simulink model "COM_Prog_Rover"  (Simulink 7.8)
settings: Solver=FixedStepDiscrete  StartTime=0.0  StopTime=inf  FixedStep=ComMinSampleTime  RelTol=1e-3
undefined symbols (not defined in the file or in its folder): ComMinSampleTime, Gumstix
settings Model: Creator=Kjenab  LastModifiedBy=keynux  ExtModeTrigDuration=10000
settings SolverCC: PositivePriorityOrder=on
settings DataIOCC: SaveFormat=StructureWithTime
settings OptimizationCC: InitFltsAndDblsToZero=on  OptimizeModelRefInitCode=on  LifeSpan=Inf
settings DebuggingCC: SaveWithParameterizedLinksMsg=none  UnderspecifiedInitializationDetection=Simplified  MergeDetectMultiDrivingBlocksExec=error  FcnCallInpInsideContextMsg=Use local settings  FrameProcessingCompatibilityMsg=error
settings RTWCC: SystemTargetFile=ert.tlc  GenCodeOnly=on  GenerateMakefile=off  TemplateMakefile=ert_default_tmf  PostCodeGenCommand=packNGo(buildInfo, {'packType' 'hierarchical'})  Description=Embedded Coder  ProcessScript=ert_make_rtw_hook
settings CodeAppCC: IgnoreCustomStorageClasses=off
settings ERTTargetCC: TargetFunctionLibrary=C89/C90 (ANSI)  MultiwordLength=2048  GenerateSampleERTMain=on  ERTCustomFileTemplate=example_file_process.tlc  ConvertIfToSwitch=off  SuppressUnreachableDefaultCases=off

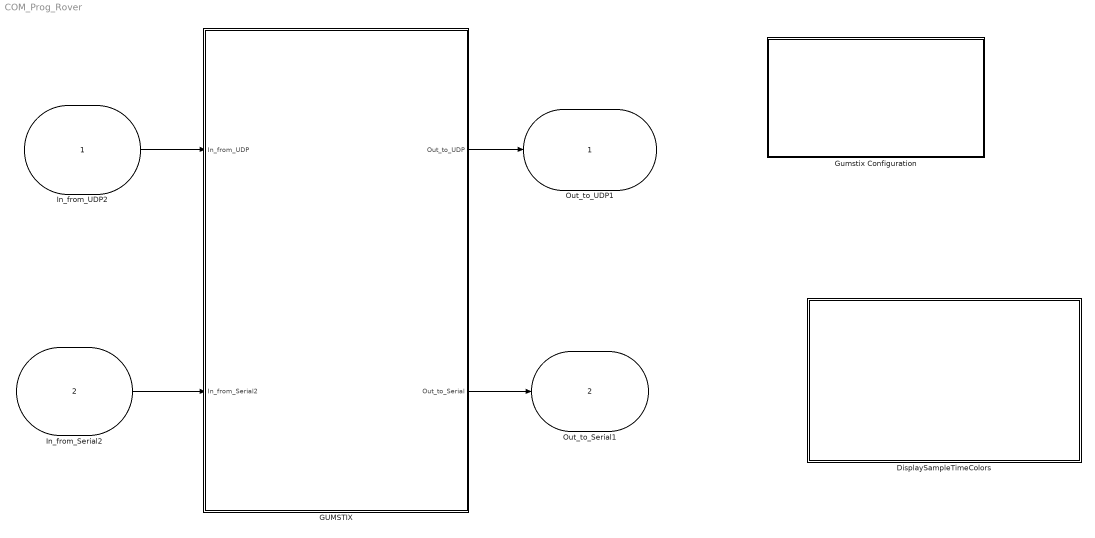
== system COM_Prog_Rover ==
  In_from_UDP2 : Inport  OutDataTypeStr=single  PortDimensions=Gumstix.UDP.Reception(1).NbData  SampleTime=Gumstix.UDP.Reception(1).SampleTime  mask{UDP_NbData=26, UDP_DataType=float32, UDP_remoteIPaddress='192.168.137.3', UDP_remotePort=2012, UDP_Interface=wlan0, UDP_localPort=2012, UDP_SampleTime=ComMinSampleTime, UDP_BlockingReception=OFF (try to read the n data), UDP_BlockingTimeOut=0.1}
      mask prompts: UDP_NbData "Number of Received Data"; UDP_DataType "UDP Data Type"; UDP_remoteIPaddress "Remote peer's IP address (IPv4)"; UDP_remotePort "Remote peer's Port (1023<port<65536)"; UDP_Interface "Local Interface to use"; UDP_localPort "Local Port (1023<port<65536)"; UDP_SampleTime "Reception Sample Time [s]"; UDP_BlockingReception "Blocking Reception"; UDP_BlockingTimeOut "Blocking Time Out [s]"
      mask init:
      | for i=1:1:8
      |     ProcessUDPInportMask_COM(gcb, i);
      | end
      mask StyleString: edit,popup(double64|float32|int32|unsigned int32|int16|unsigned int16|char8|unsigned char8),edit,edit,popup(wlan0|eth0),edit,edit,popup(ON (wait the n data until the Time Out)|OFF (try to read the n data)),edit
      mask CallbackString: ProcessUDPInportMask_COM(gcb, 1);|ProcessUDPInportMask_COM(gcb, 2);|ProcessUDPInportMask_COM(gcb, 3);|ProcessUDPInportMask_COM(gcb, 4);|ProcessUDPInportMask_COM(gcb, 5);|ProcessUDPInportMask_COM(gcb, 6);|ProcessUDPInportMask_COM(gcb, 7);|ProcessUDPInportMask_COM(gcb, 8);|ProcessUDPInportMask_COM(gcb, 9);
      mask Display: Display_UDP_Reception_Block;
  In_from_Serial2 : Inport  Port=2  OutDataTypeStr=uint8  PortDimensions=Gumstix.RS232.Reception(1).NbData  SampleTime=Gumstix.RS232.Reception(1).SampleTime  mask{RS232_NbData=6, RS232_DataType=unsigned char8, RS232_Port=/dev/ttyO0, RS232_BaudRate=115200, RS232_SampleTime=0.01, RS232_BlockingReception=OFF (try to read the n data), RS232_BlockingTimeOut=0.00022, RS232_StreamHeaderReception=1 byte, RS232_StreamHeaderValue=174, RS232_StartProtocol=SendStart -> WaitStart, RS232_StartTimeOut=100, RS232_StartStream=START, RS232_StopProtocol=None, RS232_StopTimeOut=100, RS232_StopStream=STOP}
      mask prompts: RS232_NbData "Number of Received Data"; RS232_DataType "RS232 Data Type"; RS232_Port "Serial Port"; RS232_BaudRate "BaudRate"; RS232_SampleTime "Reception Sample Time [s]"; RS232_BlockingReception "Blocking Reception"; RS232_BlockingTimeOut "Blocking Time Out [s]"; RS232_StreamHeaderReception "Stream Header"; RS232_StreamHeaderValue "Stream header value [0-255]"; RS232_StartProtocol "START Protocols"; RS232_StartTimeOut "Start Stream Waiting TimeOut [ms]"; RS232_StartStream "Start Message"; RS232_StopProtocol "STOP Protocols"; RS232_StopTimeOut "Stop Stream Waiting TimeOut [ms]"; RS232_StopStream "Stop Message"
      mask init:
      | for i=1:1:15
      |     ProcessRS232InportMask_COM(gcb, i);
      | end
      mask StyleString: edit,popup(double64|float32|int32|unsigned int32|int16|unsigned int16|char8|unsigned char8),popup(/dev/ttyO0|/dev/ttyO1|/dev/ttyO2|/dev/ttyO3|/dev/ttyO4|/dev/ttyO5|/dev/ttyO6|/dev/ttyO7|/dev/ttyO8|/dev/ttyO9|/dev/ttyO10|/dev/ttyO11|/dev/ttyO12|/dev/ttyO13|/dev/ttyO14|/dev/ttyO15|/dev/ttyUSB0|/dev/ttyUSB1),popup(50|75|110|134|150|200|300|600|1200|1800|2400|4800|9600|19200|38400|57600|115200|230400|460800|576000|921600|1000000|1152000|1500000|2000000|2500000|3000000|3500000|4000000),edit,popup(ON (wait the n data)|OFF (try to read the n data)),edit,popup(None|1 byte),edit,popup(WaitStart -> SendStart|SendStart -> WaitStart|None),edit,edit,popup(WaitStop -> SendStop|SendStop -> WaitStop|None),edit,edit
      mask CallbackString:
      | ProcessRS232InportMask_COM(gcb, 1);
      | |ProcessRS232InportMask_COM(gcb, 2);
      | |ProcessRS232InportMask_COM(gcb, 3);
      | |ProcessRS232InportMask_COM(gcb, 4);
      | |ProcessRS232InportMask_COM(gcb, 5);
      | |ProcessRS232InportMask_COM(gcb, 6);
      | |ProcessRS232InportMask_COM(gcb, 7);|ProcessRS232InportMask_COM(gcb, 8);|ProcessRS232InportMask_COM(gcb, 9);|ProcessRS232InportMask_COM(gcb, 10);
      | |ProcessRS232InportMask_COM(gcb, 11);
      | |ProcessRS232InportMask_COM(gcb, 12);
      | |ProcessRS232InportMask_COM(gcb, 13);
      | |ProcessRS232InportMask_COM(gcb, 14);
      | |ProcessRS232InportMask_COM(gcb, 15);
      mask TabNameString: Reception,Reception,Reception,Reception,Reception,Reception,Reception,Header and Synchro Protocol,Header and Synchro Protocol,Header and Synchro Protocol,Header and Synchro Protocol,Header and Synchro Protocol,Header and Synchro Protocol,Header and Synchro Protocol,Header and Synchro Protocol
      mask Display: Display_RS232_Reception_Block;
  DisplaySampleTimeColors : Subsystem  mask{SampleTime_1=0.002, SampleTime_2=0.004, SampleTime_3=0.01}
      settings: OpenFcn=DisplaySampleTimeColors;
      mask Display:
      | ColorOrder = {'red', 'green', 'blue', 'orange', 'magenta', 'gray', 'cyan', 'yellow'};
      | MyMaskPrompt =  get_param(gcb, 'MaskPrompts');
      | Nb_Prompt = length(MyMaskPrompt);
      | color('black');
      | disp(sprintf('Display Sample Time Colors\n(double-click)'));
      | offset = '\n\n';
      | for nb_line=1:1:Nb_Prompt-1
      |     offset = [offset '\n\n'];
      |     color(ColorOrder{nb_line});
      |     currentSampleTime = eval(['SampleTime_' num2str(nb_line)]);
      |     if (currentSampleTime == '0') % their is continous states
      |         eval(['disp([sprintf(offset) ''SampleTime_'' num2str(nb_line) '' (fundamental solver step) '' '' = '' num2str(SampleTime_' num2str(nb_line+1) ') ''[s] (continous states)'']);']);
      |     else
      |         if (nb_line == 1)
      |             eval(['disp([sprintf(offset) ''SampleTime_'' num2str(nb_line) '' (fundamental solver step) '' '' = '' num2str(SampleTime_' num2str(nb_line) ') ''[s]'']);']);
      |         else
      |             eval(['disp([sprintf(offset) ''SampleTime_'' num2str(nb_line) '' = '' num2str(SampleTime_' num2str(nb_line) ') ''[s]'']);']);
      |         end
      |     end
      | end
      | color('black');
      | disp([sprintf(offset) sprintf('\n\nMore than 1 SampleTime (inside)')]);
  GUMSTIX : Subsystem
  Gumstix Configuration : Subsystem  mask{TimeSynchro=Internal Clock, RS232_InterruptSource=/dev/ttyO0, UDP_InterruptSource=wlan0, PrintfMode=off, FprintfMode=off, TimeLoggerMode=off, PrintfTimeMode=off, FprintfTimeMode=off, TaskingMode=Multi-Tasking, SchedPolicy=SCHED_RR        (Real-Time Scheduler), MaxTaskPriority=96, RTsystem=PREEMPT-RT}
      mask prompts: TimeSynchro "Time Scheduler"; RS232_InterruptSource "RS232 Interrupt Source"; UDP_InterruptSource "UDP Interrupt Source"; PrintfMode "Verbose mode activated in the Gumstix console"; FprintfMode "Verbose mode logged in a file (onto Gumstix)"; TimeLoggerMode "Time logger mode activated (log time exec of each task)"; PrintfTimeMode "Execution time plotted in the Gumstix console"; FprintfTimeMode "Execution time logged in a file (onto Gumstix)"; TaskingMode "Tasking Mode"; SchedPolicy "Scheduler Policy"; MaxTaskPriority "Maximum Task Priority [1-99]"; RTsystem "RT system"
      mask init:
      | for i=1:1:12
      |     ProcessConfigMask_COM(gcb, i);
      | end
      mask StyleString: popup(RS232 Reception|Internal Clock|UDP Reception),popup(/dev/ttyS0|/dev/ttyS1|/dev/ttyS2|/dev/ttyS3|/dev/ttyO0|/dev/ttyO1|/dev/ttyO2|/dev/ttyO3),popup(wlan0|eth0),popup(off|on),popup(off|on),popup(off|on),popup(off|on),popup(off|on),popup(Multi-Tasking|Single-Tasking),popup(SCHED_FIFO     (Real-Time Scheduler)|SCHED_RR        (Real-Time Scheduler)|SCHED_OTHER (NO Real-Time Scheduler)),edit,popup(PREEMPT-RT|XENOMAI)
      mask CallbackString: ProcessConfigMask_COM(gcb, 1);|ProcessConfigMask_COM(gcb, 2);|ProcessConfigMask_COM(gcb, 3);|ProcessConfigMask_COM(gcb, 4);|ProcessConfigMask_COM(gcb, 5);|ProcessConfigMask_COM(gcb, 6);|ProcessConfigMask_COM(gcb, 7);|ProcessConfigMask_COM(gcb, 8);|ProcessConfigMask_COM(gcb, 9);|ProcessConfigMask_COM(gcb, 10);|ProcessConfigMask_COM(gcb, 11);|ProcessConfigMask_COM(gcb, 12);
      mask TabNameString: TimeScheduler,TimeScheduler,TimeScheduler,Input-Ouput Verbose,Input-Ouput Verbose,Input-Ouput Verbose,Timing Debug,Timing Debug,TimeScheduler,TimeScheduler,TimeScheduler,TimeScheduler
      mask Display: image(imread('Configuration_v2.jpg'));
  Out_to_UDP1 : Outport  OutDataTypeStr=single  PortDimensions=Gumstix.UDP.Emission(1).NbData  SampleTime=Gumstix.UDP.Emission(1).SampleTime  mask{UDP_NbData=20, UDP_DataType=float32, UDP_RemoteIPaddress='192.168.137.3', UDP_RemotePort=2012, UDP_Interface=wlan0, UDP_LocalPort=2012, UDP_SampleTime=ComMinSampleTime}
      mask prompts: UDP_NbData "Number of Sent Data"; UDP_DataType "UDP Data Type"; UDP_RemoteIPaddress "remote peer's IP address (IPv4)"; UDP_RemotePort "remote peer's Port (1023<port<65536)"; UDP_Interface "Local Interface to use for UDP"; UDP_LocalPort "Local port to use"; UDP_SampleTime "Emission Sample Time [s]"
      mask init:
      | for i=1:1:7
      |     ProcessUDPOutportMask_COM(gcb, i);
      | end
      mask StyleString: edit,popup(double64|float32|int32|unsigned int32|int16|unsigned int16|char8|unsigned char8),edit,edit,popup(wlan0|eth0),edit,edit
      mask CallbackString: ProcessUDPOutportMask_COM(gcb, 1);|ProcessUDPOutportMask_COM(gcb, 2);|ProcessUDPOutportMask_COM(gcb, 3);|ProcessUDPOutportMask_COM(gcb, 4);|ProcessUDPOutportMask_COM(gcb, 5);|ProcessUDPOutportMask_COM(gcb, 6);|ProcessUDPOutportMask_COM(gcb, 7);
      mask Display: Display_UDP_Emission_Block;
  Out_to_Serial1 : Outport  Port=2  OutDataTypeStr=uint16  PortDimensions=Gumstix.RS232.Emission(1).NbData  SampleTime=Gumstix.RS232.Emission(1).SampleTime  mask{RS232_NbData=1, RS232_DataType=unsigned int16, RS232_Port=/dev/ttyO0, RS232_BaudRate=115200, RS232_SampleTime=0.01, RS232_StreamHeaderReception=1 byte, RS232_StreamHeaderValue=174, RS232_StartProtocol=SendStart -> WaitStart, RS232_StartTimeOut=100, RS232_StartStream=START, RS232_StopProtocol=None, RS232_StopTimeOut=100, RS232_StopStream=STOP}
      mask prompts: RS232_NbData "Number of Sent Data"; RS232_DataType "RS232 Data Type"; RS232_Port "Serial Port"; RS232_BaudRate "BaudRate"; RS232_SampleTime "Sample Time [s]"; RS232_StreamHeaderReception "Stream Header"; RS232_StreamHeaderValue "Stream header value [0-255]"; RS232_StartProtocol "RS232 Start Protocol"; RS232_StartTimeOut "Start Stream Waiting TimeOut [ms]"; RS232_StartStream "Start Message"; RS232_StopProtocol "RS232 Stop Protocol"; RS232_StopTimeOut "Stop Stream Waiting TimeOut [ms]"; RS232_StopStream "Stop Message"
      mask init:
      | for i=1:1:13
      |     ProcessRS232OutportMask_COM(gcb, i);
      | end
      mask StyleString: edit,popup(double64|float32|int32|unsigned int32|int16|unsigned int16|char8|unsigned char8),popup(/dev/ttyO0|/dev/ttyO1|/dev/ttyO2|/dev/ttyO3|/dev/ttyO4|/dev/ttyO5|/dev/ttyO6|/dev/ttyO7|/dev/ttyO8|/dev/ttyO9|/dev/ttyO10|/dev/ttyO11|/dev/ttyO12|/dev/ttyO13|/dev/ttyO14|/dev/ttyO15|/dev/ttyUSB0|/dev/ttyUSB1),popup(50|75|110|134|150|200|300|600|1200|1800|2400|4800|9600|19200|38400|57600|115200|230400|460800|576000|921600|1000000|1152000|1500000|2000000|2500000|3000000|3500000|4000000),edit,popup(None|1 byte),edit,popup(WaitStart -> SendStart|SendStart -> WaitStart|None),edit,edit,popup(WaitStop -> SendStop|SendStop -> WaitStop|None),edit,edit
      mask CallbackString:
      | ProcessRS232OutportMask_COM(gcb, 1);
      | |ProcessRS232OutportMask_COM(gcb, 2);
      | |ProcessRS232OutportMask_COM(gcb, 3);
      | |ProcessRS232OutportMask_COM(gcb, 4);
      | |ProcessRS232OutportMask_COM(gcb, 5);
      | |ProcessRS232OutportMask_COM(gcb, 6);|ProcessRS232OutportMask_COM(gcb, 7);|ProcessRS232OutportMask_COM(gcb, 8);|ProcessRS232OutportMask_COM(gcb, 9);|ProcessRS232OutportMask_COM(gcb, 10);|ProcessRS232OutportMask_COM(gcb, 11);|ProcessRS232OutportMask_COM(gcb, 12);|ProcessRS232OutportMask_COM(gcb, 13);
      mask TabNameString: Emission,Emission,Emission,Emission,Emission,Header and Synchro Protocol,Header and Synchro Protocol,Header and Synchro Protocol,Header and Synchro Protocol,Header and Synchro Protocol,Header and Synchro Protocol,Header and Synchro Protocol,Header and Synchro Protocol
      mask Display: Display_RS232_Emission_Block;
  wires:
  GUMSTIX/1(Out_to_UDP) -> Out_to_UDP1/1
  In_from_UDP2/1 -> GUMSTIX/1(In_from_UDP)
  In_from_Serial2/1 -> GUMSTIX/2("In_from_Serial2 ")
  GUMSTIX/2(Out_to_Serial) -> Out_to_Serial1/1

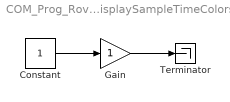
== system COM_Prog_Rover/DisplaySampleTimeColors ==
  Constant : Constant  OutDataTypeStr=uint8
  Gain : Gain
  Terminator : Terminator
  wires:
  Constant/1 -> Gain/1
  Gain/1 -> Terminator/1

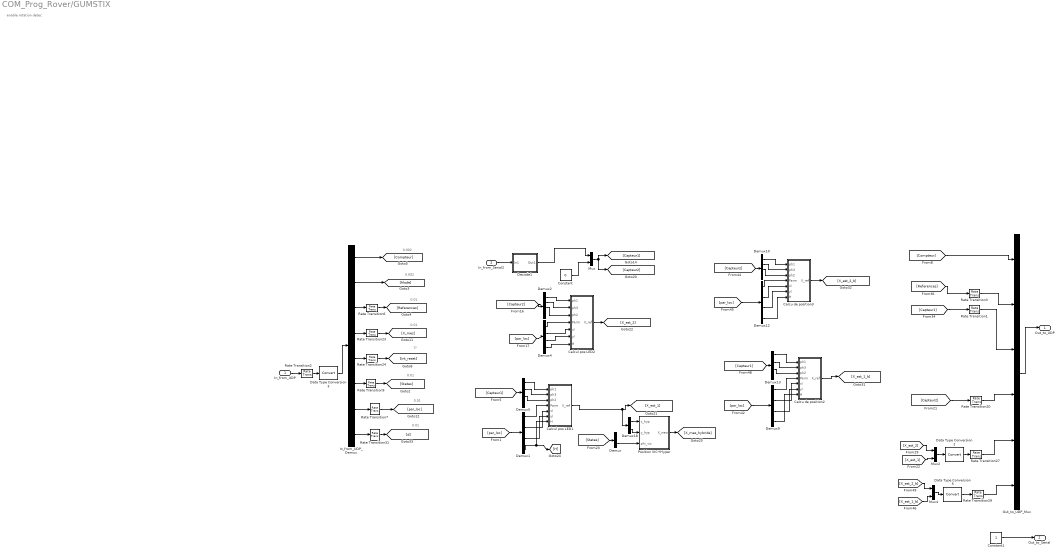
== system COM_Prog_Rover/GUMSTIX ==
  note: enable rotation detec
  note: 0.002
  note: 0.002
  note: 0.01
  note: 0.01
  note: 0.01
  note: 0.01
  note: 0.01
  note: ??
  In_from_UDP : Inport
  "In_from_Serial2 " : Inport  Port=2
  Calcu de position2 : MATLAB Function  TreatAsAtomicUnit=on
  Calcu de position3 : MATLAB Function  TreatAsAtomicUnit=on
  Calcul pos LED1 : MATLAB Function  TreatAsAtomicUnit=on
  Calcul pos LED2 : MATLAB Function  TreatAsAtomicUnit=on
  Constant : Constant  Value=0  OutDataTypeStr=Inherit: Inherit via back propagation  SampleTime=0.01
  Constant1 : Constant  OutDataTypeStr=Inherit: Inherit via back propagation  SampleTime=0.01
  Data Type Conversion2 : DataTypeConversion
  Data Type Conversion3 : DataTypeConversion
  Data Type Conversion5 : DataTypeConversion
  Decode1 : Subsystem
  Demux : Demux  Outputs=[2 1]
  Demux{1,4,9,12} (4 alike) : Demux  Outputs=[10 1 1 1]
  Demux10 : Demux  Outputs=[ 1 1 1 1]
  Demux13 : Demux  Outputs=[ 1 1 1 1]
  Demux18 : Demux  Outputs=[1 1]
  Demux2 : Demux  Outputs=[1 1 1 1]
  Demux5 : Demux  Outputs=[1 1 1 1]
  In_from_UDP_Demux : Demux  Outputs=[1 1 3 3 1 3 13 1]
  Mux : Mux  Inputs=2
  Mux2 : Mux  Inputs=2
  Mux4 : Mux  Inputs=2
  Out_to_UDP_Mux : Mux  Inputs=[1 3 4 4 4 4]
  Position VIC+Hyper : MATLAB Function  TreatAsAtomicUnit=on
  Rate Transition{1,3,20,27,29} (5 alike) : RateTransition
  Rate Transition2 : RateTransition  Deterministic=off
  Rate Transition{6..7,9,23,31} (5 alike) : RateTransition  Deterministic=off  OutPortSampleTime=Ts_control
  Rate Transition24 : RateTransition  Deterministic=off
  Out_to_UDP : Outport
  Out_to_Serial : Outport  Port=2
  wires:
  In_from_UDP/1 -> Rate Transition2/1
  Rate Transition2/1 -> Data Type Conversion3/1
  Data Type Conversion3/1 -> In_from_UDP_Demux/1
  In_from_UDP_Demux/1 -> [Compteur]
  In_from_UDP_Demux/2 -> [Mode]
  Rate Transition9/1 -> [States]
  [References] -> Rate Transition3/1
  Rate Transition6/1 -> [References]
  Rate Transition23/1 -> [X_mes]
  Rate Transition24/1 -> [Int_reset]
  Rate Transition3/1 -> Out_to_UDP_Mux/2
  Demux1/1 -> Calcul pos LED1/4(Parm)
  Rate Transition7/1 -> [par_loc]
  Demux1/2 -> Calcul pos LED1/5(xl)
  Demux1/3 -> Calcul pos LED1/6(yl)
  Demux1/4 -> [H], Calcul pos LED1/7(H)
  [Capteur2] -> Rate Transition20/1
  [par_loc] -> Demux4/1
  Demux4/1 -> Calcul pos LED2/4(Parm)
  Demux4/2 -> Calcul pos LED2/5(xl)
  Demux4/3 -> Calcul pos LED2/6(yl)
  Demux4/4 -> Calcul pos LED2/7(H)
  [Capteur2] -> Demux2/1
  Calcul pos LED2/1(X_ref) -> [X_est_2]
  [Compteur] -> Out_to_UDP_Mux/1
  Out_to_UDP_Mux/1 -> Out_to_UDP/1
  [X_est_2] -> Mux2/1
  Mux2/1 -> Data Type Conversion2/1
  Data Type Conversion2/1 -> Rate Transition27/1
  [X_est_1] -> Mux2/2
  Position VIC+Hyper/1(X_new) -> [X_mes_hybride]
  [Capteur1] -> Rate Transition1/1
  [States] -> Demux/1
  Demux9/1 -> Calcu de position2/4(Parm)
  [par_loc] -> Demux9/1
  Demux9/2 -> Calcu de position2/5(xl)
  Demux9/3 -> Calcu de position2/6(yl)
  Demux9/4 -> Calcu de position2/7(H)
  [Capteur1] -> Demux13/1
  [par_loc] -> Demux12/1
  Demux12/1 -> Calcu de position3/4(Parm)
  Demux12/2 -> Calcu de position3/5(xl)
  Demux12/3 -> Calcu de position3/6(yl)
  Demux12/4 -> Calcu de position3/7(H)
  [Capteur2] -> Demux10/1
  Calcu de position3/1(X_ref) -> [X_est_2_b]
  Demux10/1 -> Calcu de position3/1(ph1)
  Demux10/2 -> Calcu de position3/2(ph3)
  Demux10/3 -> Calcu de position3/3(ph2)
  Demux13/1 -> Calcu de position2/1(ph1)
  Demux13/2 -> Calcu de position2/2(ph3)
  Demux13/3 -> Calcu de position2/3(ph2)
  Calcul pos LED1/1(X_ref) -> Demux18/1, [X_est_1]
  [X_est_2_b] -> Mux4/1
  Mux4/1 -> Data Type Conversion5/1
  Data Type Conversion5/1 -> Rate Transition29/1
  [X_est_1_b] -> Mux4/2
  Rate Transition31/1 -> [d]
  Demux18/2 -> Position VIC+Hyper/2(y_hyp)
  Demux18/1 -> Position VIC+Hyper/1(x_hyp)
  Demux/2 -> Position VIC+Hyper/3(phi_vic)
  [par_loc] -> Demux1/1
  [Capteur1] -> Demux5/1
  Calcu de position2/1(X_ref) -> [X_est_1_b]
  Rate Transition1/1 -> Out_to_UDP_Mux/3
  In_from_UDP_Demux/3 -> Rate Transition6/1
  In_from_UDP_Demux/4 -> Rate Transition23/1
  In_from_UDP_Demux/5 -> Rate Transition24/1
  In_from_UDP_Demux/6 -> Rate Transition9/1
  In_from_UDP_Demux/7 -> Rate Transition7/1
  In_from_UDP_Demux/8 -> Rate Transition31/1
  Rate Transition20/1 -> Out_to_UDP_Mux/4
  Rate Transition27/1 -> Out_to_UDP_Mux/5
  Rate Transition29/1 -> Out_to_UDP_Mux/6
  "In_from_Serial2 "/1 -> Decode1/1(In1)
  Decode1/1(Out1) -> Mux/1
  Constant/1 -> Mux/2
  Mux/1 -> [Capteur1], [Capteur2]
  Demux2/1 -> Calcul pos LED2/1(ph1)
  Demux2/2 -> Calcul pos LED2/2(ph3)
  Demux2/3 -> Calcul pos LED2/3(ph2)
  Demux5/1 -> Calcul pos LED1/1(ph1)
  Demux5/2 -> Calcul pos LED1/2(ph3)
  Demux5/3 -> Calcul pos LED1/3(ph2)
  Constant1/1 -> Out_to_Serial/1

== system COM_Prog_Rover/Gumstix Configuration ==

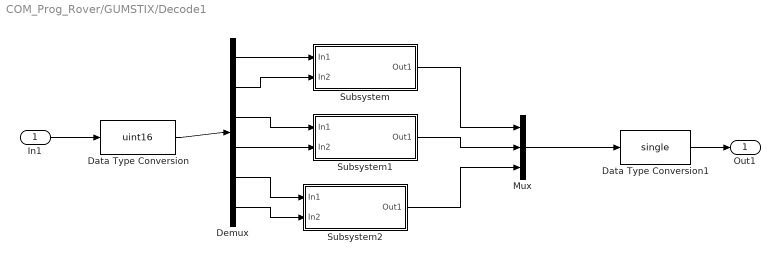
== system COM_Prog_Rover/GUMSTIX/Decode1 ==
  In1 : Inport
  Data Type Conversion : DataTypeConversion  OutDataTypeStr=uint16
  Data Type Conversion1 : DataTypeConversion  OutDataTypeStr=single
  Demux : Demux  Outputs=6
  Mux : Mux  Inputs=3
  Subsystem : Subsystem
  Subsystem1 : Subsystem
  Subsystem2 : Subsystem
  Out1 : Outport
  wires:
  Data Type Conversion1/1 -> Out1/1
  In1/1 -> Data Type Conversion/1
  Data Type Conversion/1 -> Demux/1
  Demux/1 -> Subsystem/1(In1)
  Demux/2 -> Subsystem/2(In2)
  Demux/3 -> Subsystem1/1(In1)
  Demux/4 -> Subsystem1/2(In2)
  Demux/5 -> Subsystem2/1(In1)
  Demux/6 -> Subsystem2/2(In2)
  Subsystem/1(Out1) -> Mux/1
  Subsystem1/1(Out1) -> Mux/2
  Subsystem2/1(Out1) -> Mux/3
  Mux/1 -> Data Type Conversion1/1

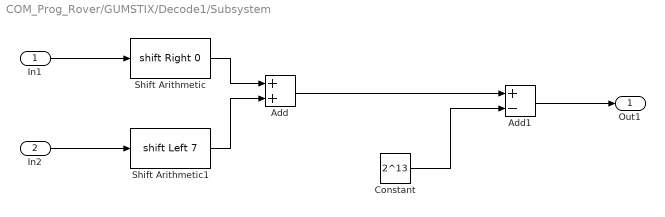
== system COM_Prog_Rover/GUMSTIX/Decode1/Subsystem ==
  In1 : Inport
  In2 : Inport  Port=2
  Add : Sum
  Add1 : Sum  Inputs=+-
  Constant : Constant  Value=2^13  OutDataTypeStr=uint16  SampleTime=-1
  Shift Arithmetic : ArithShift  BitShiftDirection=Right
  Shift Arithmetic1 : ArithShift  BitShiftNumber=7  BitShiftDirection=Left
  Out1 : Outport
  wires:
  In1/1 -> Shift Arithmetic/1
  In2/1 -> Shift Arithmetic1/1
  Shift Arithmetic/1 -> Add/1
  Shift Arithmetic1/1 -> Add/2
  Add/1 -> Add1/1
  Constant/1 -> Add1/2
  Add1/1 -> Out1/1

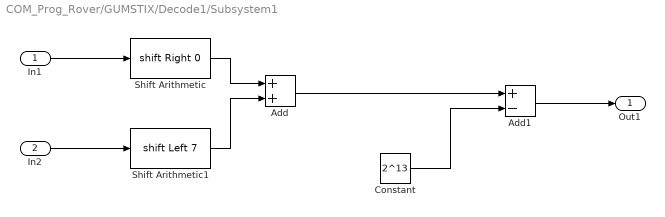
== system COM_Prog_Rover/GUMSTIX/Decode1/Subsystem1 ==
  In1 : Inport
  In2 : Inport  Port=2
  Add : Sum
  Add1 : Sum  Inputs=+-
  Constant : Constant  Value=2^13  OutDataTypeStr=uint16  SampleTime=-1
  Shift Arithmetic : ArithShift  BitShiftDirection=Right
  Shift Arithmetic1 : ArithShift  BitShiftNumber=7  BitShiftDirection=Left
  Out1 : Outport
  wires:
  In1/1 -> Shift Arithmetic/1
  In2/1 -> Shift Arithmetic1/1
  Shift Arithmetic/1 -> Add/1
  Shift Arithmetic1/1 -> Add/2
  Add/1 -> Add1/1
  Constant/1 -> Add1/2
  Add1/1 -> Out1/1

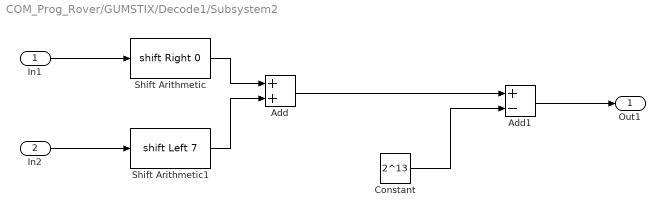
== system COM_Prog_Rover/GUMSTIX/Decode1/Subsystem2 ==
  In1 : Inport
  In2 : Inport  Port=2
  Add : Sum
  Add1 : Sum  Inputs=+-
  Constant : Constant  Value=2^13  OutDataTypeStr=uint16  SampleTime=-1
  Shift Arithmetic : ArithShift  BitShiftDirection=Right
  Shift Arithmetic1 : ArithShift  BitShiftNumber=7  BitShiftDirection=Left
  Out1 : Outport
  wires:
  In1/1 -> Shift Arithmetic/1
  In2/1 -> Shift Arithmetic1/1
  Shift Arithmetic/1 -> Add/1
  Shift Arithmetic1/1 -> Add/2
  Add/1 -> Add1/1
  Constant/1 -> Add1/2
  Add1/1 -> Out1/1

== matlab function GUMSTIX/Calcul pos LED2 ==
  data: ph1 input double; ph3 input double; X_ref output double; ph2 input double; Parm input double; xl input double; yl input double; H input double
function X_ref = position(ph1, ph3, ph2, Parm, xl, yl, H)   %xl,yl,H qre position of LED1
trd = pi/180;
tr2 = (ph1-ph2)/(ph1+ph2);
tr1 = (((ph1+ph2)/2)-ph3)/(((ph1+ph2)/2)+ph3);
%x = H*tan(trd*(a1*tr1+b1));
%y = H*tan(trd*(a2*tr2+b2));
% x = H.*tan(trd.*(Parm(1).*tr1 + Parm(2).*tr1.^2+ Parm(3).*tr2+Parm(4) ));
% y = H.*tan(trd.*(Parm(5).*tr2 + Parm(6).*tr2.^2+Parm(7).*tr1 + Parm(8)));
x = H.*tan(trd.*(Parm(1).*tr1 + Parm(2).*tr1.^2+ Parm(3).*tr2+  Parm(4).*tr2.^2+Parm(5) ));
y = H.*tan(trd.*(Parm(6).*tr2 + Parm(7).*tr2.^2+Parm(8).*tr1 + Parm(9).*tr1.^2+Parm(10)));
X_ref = [x,y];
end

== matlab function GUMSTIX/Calcu de position2 ==
  data: ph1 input double; ph3 input double; X_ref output double; ph2 input double; Parm input double; xl input double; yl input double; H input double
function X_ref = position(ph1, ph3, ph2, Parm, xl, yl, H)
trd = pi/180;
tr2 = (ph1-ph2)/(ph1+ph2);
tr1 = (((ph1+ph2)/2)-ph3)/(((ph1+ph2)/2)+ph3);
%x = H*tan(trd*(a1*tr1+b1));
%y = H*tan(trd*(a2*tr2+b2));
% x = H.*tan(trd.*(Parm(1).*tr1 + Parm(2).*tr1.^2+ Parm(3).*tr2+Parm(4) ));
% y = H.*tan(trd.*(Parm(5).*tr2 + Parm(6).*tr2.^2+Parm(7).*tr1 + Parm(8)));
x = H.*tan(trd.*(Parm(1).*tr1 + Parm(2).*tr1.^2+ Parm(3).*tr2+  Parm(4).*tr2.^2+Parm(5) ));
y = H.*tan(trd.*(Parm(6).*tr2 + Parm(7).*tr2.^2+Parm(8).*tr1 + Parm(9).*tr1.^2+Parm(10)));
X_ref = [x,y];
end

== matlab function GUMSTIX/Calcul pos LED1 ==
  data: ph1 input double; ph3 input double; X_ref output double; ph2 input double; Parm input double; xl input double; yl input double; H input double
function X_ref = position(ph1, ph3, ph2, Parm, xl, yl, H)
trd = pi/180;
tr2 = (ph1-ph2)/(ph1+ph2);
tr1 = (((ph1+ph2)/2)-ph3)/(((ph1+ph2)/2)+ph3);
%x = H*tan(trd*(a1*tr1+b1));
%y = H*tan(trd*(a2*tr2+b2));
% x = H.*tan(trd.*(Parm(1).*tr1 + Parm(2).*tr1.^2+ Parm(3).*tr2+Parm(4) ));
% y = H.*tan(trd.*(Parm(5).*tr2 + Parm(6).*tr2.^2+Parm(7).*tr1 + Parm(8)));
x = H.*tan(trd.*(Parm(1).*tr1 + Parm(2).*tr1.^2+ Parm(3).*tr2+  Parm(4).*tr2.^2+Parm(5) ));
y = H.*tan(trd.*(Parm(6).*tr2 + Parm(7).*tr2.^2+Parm(8).*tr1 + Parm(9).*tr1.^2+Parm(10)));
X_ref = [x,y];
end

== matlab function GUMSTIX/Calcu de position3 ==
  data: ph1 input double; ph3 input double; X_ref output double; ph2 input double; Parm input double; xl input double; yl input double; H input double
function X_ref = position(ph1, ph3, ph2, Parm, xl, yl, H)
trd = pi/180;
tr2 = (ph1-ph2)/(ph1+ph2);
tr1 = (((ph1+ph2)/2)-ph3)/(((ph1+ph2)/2)+ph3);
%x = H*tan(trd*(a1*tr1+b1));
%y = H*tan(trd*(a2*tr2+b2));
% x = H.*tan(trd.*(Parm(1).*tr1 + Parm(2).*tr1.^2+ Parm(3).*tr2+Parm(4) ));
% y = H.*tan(trd.*(Parm(5).*tr2 + Parm(6).*tr2.^2+Parm(7).*tr1 + Parm(8)));
x = H.*tan(trd.*(Parm(1).*tr1 + Parm(2).*tr1.^2+ Parm(3).*tr2+  Parm(4).*tr2.^2+Parm(5) ));
y = H.*tan(trd.*(Parm(6).*tr2 + Parm(7).*tr2.^2+Parm(8).*tr1 + Parm(9).*tr1.^2+Parm(10)));
X_ref = [x,y];
end

== matlab function GUMSTIX/Position VIC+Hyper ==
  data: x_hyp input double; y_hyp input double; X_new output double; phi_vic input double
function X_new = position(x_hyp, y_hyp, phi_vic)
phi = phi_vic;
A = [cos(phi) -sin(phi) 0; sin(phi) cos(phi) 0; 0 0 1];
X = A*[x_hyp;y_hyp;phi_vic];
X_new = X';
end
